simulink model "MotoTron_validation_IO_model_integration"  (R2018a)
settings: Solver=FixedStepDiscrete  StartTime=0.0  StopTime=10.0  RelTol=1e-3  EnableMultiTasking=on
undefined symbols (not defined in the file or in its folder): ECU565, motohawk_build_version, motohawk_trunc_name, motohawk_vardec_path
libraries: MotoHawk_lib x73, simulink x16, motohawk_examples_lib x1
(part 1 of 2)
settings Model: MotoHawkModelGUID=81168908-1F61-4548-B973-A09766F2E4F2  MotoHawkModelOpenTime=2019 4 16 12 38 3.57  MotoHawkBuildVersion=001  MotoHawkBuildStats=struct('TotalFLASH',{0},'TotalEEPROM',{0},'TotalRAM',{0},'AppFLASH',{0},'AppEEPROM',{0},'AppRAM',{0},'HeapRAM',{0},'BuildSuccessCount',{1},'BuildErrorCount',{0})  MotoHawkBuildDirectory=C:\Users\dhruv\OneDrive\Desktop\MEEM 5750\Project_Final5750\MotoTron_validation_IO_model_integration_Build  MotoHawkBuildInfo=struct('refmodel',{0},'model_name',{'MotoTron_validation_IO_model_2019'},'motohawk_version',{'2018a_sp2.2221'},'motohawk_component_version',{'0.0.8'},'motohawk_refmdl_version',{'0.0.1'},'matlab_version',{'9.4.0'},'build_version',{'000'},'module_type',{'ECU565-128'},'layout_type',{'DEV'},'enable_build',{1},'processor_family',{'PPC'},'processor_type',{'MPC565'},'toolchain_vendor',{'gcc-powerpc-eabi'},'toolchain_version',{'4.6.0'},'component',{0},'archive_file',{'PCM128.a'},'fptype',{0},'flash_size',{1048576},'ee_size',{8192},'ram_size',{36864},'decram_size',{4096},'eri_table0_rev',{12},'max_eri_table_size',{65535},'fgnd_base_period_ms',{5},'bgnd_base_period_ms',{50},'build_dir',{'D:\Slides\MotoTron_validation_IO_model_2019_Build'},'dll_name',{'MotoTron_validation_IO_model_2019_000'},'srz_name',{'MotoTron_validation_IO_model_2019_000'},'fgnd_stack_size',{3072},'fgnd_angle_stack_size',{0},'bgnd_stack_size',{2048},'idle_stack_size',{1024},'irq_stack_size',{1536},'irq_stack_margin',{153},'heap_size',{4096},'heap_margin',{409},'app_int_stack_size',{1024},'shutdown_stack_size',{1024},'use_target_os_config',{0},'num_cores_in_use',{1},'target_os',{'Classic ControlCore'},'install_dll_dir',{'C:\ECUFiles\TDBDLL'},'install_srz_dir',{'C:\ECUFiles\Programs'},'mingw_dir',{'C:\Program Files (x86)\Woodward\DevelopmentTools\Toolchains\GCC\win64-pe\4_7_1'},'motohawk_dir',{'C:\Program Files (x86)\Woodward\MCS\MotoHawk\2018a_sp2.2221'},'toolchain_dir',{'C:\Program Files (x86)\Woodward\DevelopmentTools\Toolchains\GCC\powerpc-eabi\4_6_0'},'matlab_root',{'C:\Program Files\MATLAB\R2018a'},'model_guid',{'030D1D23-8488-4897-A5F8-BE99CB1E4A09'},'build_guid',{'2DCC9D67-0315-4B80-8A59-7423BF9FA0F1'},'token_guid',{'26AE92E680E3264698612664E4C57D6C'})  MotoHawkModelSavedName=MotoTron_validation_IO_model_integration  MotoHawkModelElapsedTime=291694.622  MotoHawkBuildGUID=2DCC9D67-0315-4B80-8A59-7423BF9FA0F1  Creator=wzhouqua  LastModifiedBy=dhruv
settings ConfigSet: Description="This Simulink Configuration Set is preconfigured  for the MotoHawk target \"ECU565-128\"."
settings OptimizationCC: DefaultParameterBehavior=Inlined  InlineInvariantSignals=on  EnhancedBackFolding=on  InitFltsAndDblsToZero=on  NoFixptDivByZeroProtection=on  EfficientFloat2IntCast=on  LifeSpan=1
settings DebuggingCC: InheritedTsInSrcMsg=none  TasksWithSamePriorityMsg=none  ModelReferenceIOMismatchMessage=warning  SFUnexpectedBacktrackingDiag=warning  SFNoUnconditionalDefaultTransitionDiag=warning  SFExecutionAtInitializationDiag=none
settings HardwareCC: ProdBitPerPointer=32  ProdBitPerSizeT=32  ProdBitPerPtrDiffT=32  ProdLargestAtomicInteger=Integer  ProdIntDivRoundTo=Undefined  ProdEndianess=BigEndian  ProdWordSize=32  ProdHWDeviceType=Specified
settings ModelReferenceCC: UpdateModelReferenceTargets=IfOutOfDate  CheckModelReferenceTargetMessage=warning  ModelReferenceNumInstancesAllowed=Single
settings SFSimCC: MATLABDynamicMemAlloc=off
settings RTWCC: SystemTargetFile=motohawk_ert_rtw.tlc  MakeCommand=make_rtw_motohawk  TemplateMakefile=motohawk_ert_rtw.tmf  Description=MotoHawk(tm) Rapid Prototyping  GenerateReport=on  IncludeHyperlinkInReport=on  LaunchReport=on  GenerateTraceInfo=on  GenerateTraceReport=on  GenerateTraceReportSl=on  GenerateTraceReportSf=on  GenerateTraceReportEml=on
settings CodeAppCC: ForceParamTrailComments=on  IgnoreCustomStorageClasses=off  MaxIdLength=100  OperatorAnnotations=on  SimulinkDataObjDesc=on  SFDataObjDesc=on  MATLABFcnDesc=on  CustomSymbolStrType=$N$R$M  CustomSymbolStrField=$H$N$M  InsertBlockDesc=on  StateflowObjectComments=on  MATLABSourceComments=on  InternalIdentifier=Classic
settings STFCustomTargetCC: MultiwordTypeDef=User defined  MultiwordLength=0  IncludeMdlTerminateFcn=off  GeneratePreprocessorConditionals=Disable all  CombineOutputUpdateFcns=on  SuppressErrorStatus=on  ERTCustomFileBanners=on  SupportContinuousTime=off  SupportNonInlinedSFcns=off  RemoveResetFunc=on  MATLABClassNameForMDSCustomization=Simulink.SoftwareTarget.ERTCustomization  GRTInterface=off  SystemTargetFile=motohawk_ert_rtw.tlc
settings ERTTargetCC: MultiwordTypeDef=User defined  MultiwordLength=0  ParMdlRefBuildCompliant=off  CompOptLevelCompliant=off  ConcurrentExecutionCompliant=off  IncludeMdlTerminateFcn=off  GeneratePreprocessorConditionals=Disable all  SuppressErrorStatus=on  ModelStepFunctionPrototypeControlCompliant=off  CPPClassGenCompliant=off  UseToolchainInfoCompliant=off  InlinedParameterPlacement=NonHierarchical  ERTCustomFileTemplate=motohawk_file_process.tlc
settings ConfigComp: CovMetricSettings=dw  CovHtmlReporting=on  CovSaveCumulativeToWorkspaceVar=on  CovSaveSingleToWorkspaceVar=on  CovExternalEMLEnable=off

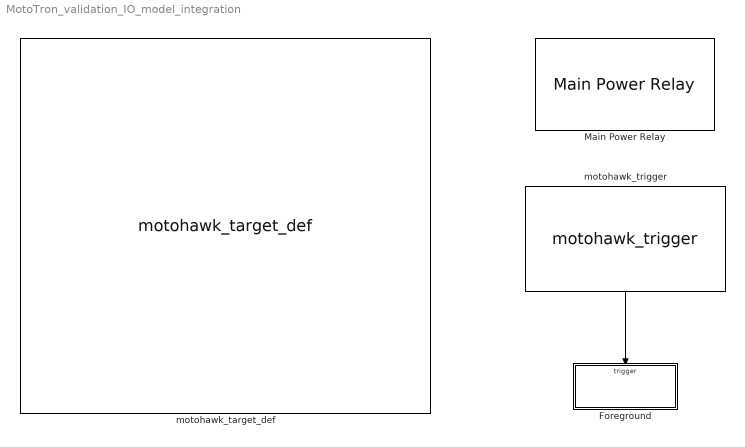
== system MotoTron_validation_IO_model_integration ==
  Foreground : Subsystem  InitFcn=data  TreatAsAtomicUnit=on
  Main Power Relay : motohawk_examples_lib/Main Power Relay Blocks/Main Power Relay  on_delay_count=2  off_delay_count=5  ecup_threshold=100  group='System | Main Power Relay'
      settings: SourceProductName=MotoHawk
  motohawk_target_def : MotoHawk_lib/motohawk_target_def  Priority=-65535  target=ECU565-128  layout=DEV  fptype=single (32 bits)  use_target_os_config=off  target_os=ControlCore  default_target_os=Classic ControlCore  fgnd_stack_size=3*1024  fgnd_angle_stack_size=0  bgnd_stack_size=2*1024  idle_stack_size=1024  irq_stack_size=1536  app_int_stack_size=1024  shutdown_stack_size=1024  heap_size=4*1024  show_margins=off  fgnd_stack_margin=(3*1024) * 0.1  fgnd_angle_stack_margin=0  bgnd_stack_margin=(2*1024) * 0.1  idle_stack_margin=(1024) * 0.1  irq_stack_margin=(1536) * 0.1  app_int_stack_margin=(1024) * 0.1  shutdown_stack_margin=(1024) * 0.1  heap_margin=(4*1024) * 0.1  comp_name=bdroot  comp_img='KVASER_CAN_USB.jpg'  comp_security=No Encryption  comp_build_pass='mhbuild'  comp_sim_pass='mhsim'  comp_multi=off  show_filenames=off  dll_name=motohawk_trunc_name(bdroot, ['_' motohawk_build_version], 50)  srz_name=motohawk_trunc_name(bdroot, ['_' motohawk_build_version], 50)  build_dir='.'  comp_dir='.'
      settings: SourceProductName=MotoHawk
  motohawk_trigger : MotoHawk_lib/Trigger Blocks/motohawk_trigger  Tag=Trigger  Priority=0  trig_name=[]  trigger=FGND_RTI_PERIODIC  priority_order=0  inherited=off  run_disabled=off  override_app_monitor=off  target=ECU565_128
      settings: SourceProductName=MotoHawk
  wires:
  motohawk_trigger/1 -> Foreground/Trigger

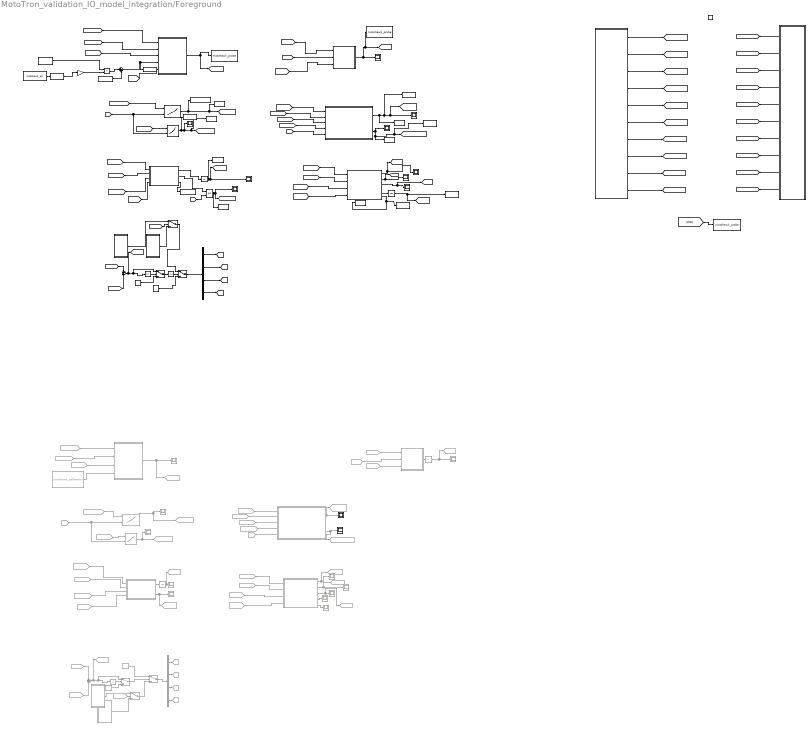
== system MotoTron_validation_IO_model_integration/Foreground ==
  note: Engine Start/Stop Model
  note: Torque Request
  note: Engine State Logic Model
  note: Blend Factor Lookup Tables
  note: StepperMotor
  note: Driving Mode Model
  note: E-Motor Start/Stop Model
  note: Blend Factor Lookup Tables
  note: Engine Start/Stop Model
  note: Driving Mode Model
  note: Engine State Logic Model
  note: StepperMotor
  note: E-Motor Start/Stop Model
  note: Torque Request
  function : TriggerPort  TriggerType=function-call  VariantControl=Variant
  2-D Lookup Table : Lookup_n-D  Commented=on  BreakpointsForDimension1=Engine_Blend_Factor(2:end,1)  BreakpointsForDimension2=Engine_Blend_Factor(1,2:end)  Table=Engine_Blend_Factor(2:end,2:end)  InternalRulePriority=Speed  RndMeth=Simplest  InputSameDT=on
  2-D Lookup Table1 : Lookup_n-D  InitFcn=data  BreakpointsForDimension1=Engine_Blend_Factor(2:end,1)  BreakpointsForDimension2=Engine_Blend_Factor(1,2:end)  Table=Engine_Blend_Factor(2:end,2:end)  InternalRulePriority=Speed  RndMeth=Simplest  InputSameDT=on
  Abs : Abs  Commented=on
  Abs1 : Abs
  Abs2 : Abs
  Actuator : Subsystem
  CCW : Subsystem  Commented=on
  CCW1 : Subsystem
  CW : Subsystem  Commented=on
  CW1 : Subsystem
  Cast : DataTypeConversion  OutDataTypeStr=double
  Chart : Stateflow chart  Commented=on  TreatAsAtomicUnit=on
  Chart1 : Stateflow chart  Commented=on  TreatAsAtomicUnit=on
  Chart2 : Stateflow chart  TreatAsAtomicUnit=on
  Chart3 : Stateflow chart  TreatAsAtomicUnit=on
  Constant : Constant  Commented=on  Value=0
  Constant1 : Constant  Commented=on  Value=0
  Constant2 : Constant  Value=0
  Constant3 : Constant  Value=0
  Demux : Demux  Commented=on
  Demux1 : Demux
  "Engine State " : Stateflow chart  Commented=on  TreatAsAtomicUnit=on
  Engine State 1 : Stateflow chart  TreatAsAtomicUnit=on
  From : From  Commented=on  GotoTag=Vehicle_Speed
  From11 : From  Commented=on  GotoTag=Vehicle_Speed
  From12 : From  Commented=on  GotoTag=motorblendfactor
  From13 : From  Commented=on  GotoTag=drivingmode
  From14 : From  Commented=on  GotoTag=engineblendfactor
  From15 : From  Commented=on  GotoTag=motorblendfactor
  From16 : From  Commented=on  GotoTag=drivingmode
  From17 : From  Commented=on  GotoTag=Engine_State
  From18 : From  Commented=on  GotoTag=PPS1
  From19 : From  Commented=on  GotoTag=engineblendfactor
  From20 : From  Commented=on  GotoTag=drivingmode
  From21 : From  Commented=on  GotoTag=Engine_State
  From22 : From  Commented=on  GotoTag=Engine_On_Switch
  From23 : From  Commented=on  GotoTag=Motor_On_Switch
  From24 : From  Commented=on  GotoTag=Vehicle_Speed
  From25 : From  Commented=on  GotoTag=Engine_RPM
  From26 : From  Commented=on  GotoTag=Crank_Switch
  From27 : From  Commented=on  GotoTag=PPS1
  From28 : From  Commented=on  GotoTag=Crank_Switch
  From29 : From  Commented=on  GotoTag=Forward_Switch
  From30 : From  Commented=on  GotoTag=Reverse_Switch
  From31 : From  Commented=on  GotoTag=enginethrottle
  From32 : From  Commented=on  GotoTag=TPS
  From33 : From  Commented=on  GotoTag=Engine_Kill
  From35 : From  Commented=on  GotoTag=difference
  Gain : Gain  Gain=5/1023
  Goto10 : Goto  Commented=on  GotoTag=Engine_State
  Goto11 : Goto  Commented=on  GotoTag=engineblendfactor
  Goto12 : Goto  Commented=on  GotoTag=motorblendfactor
  Goto13 : Goto  Commented=on  GotoTag=E_Motor_Toruqe_Request
  Goto14 : Goto  Commented=on  GotoTag=Forward
  Goto15 : Goto  Commented=on  GotoTag=enginethrottle
  Goto16 : Goto  Commented=on  GotoTag=Coil_4
  Goto17 : Goto  Commented=on  GotoTag=Coil_1
  Goto18 : Goto  Commented=on  GotoTag=Coil_2
  Goto19 : Goto  Commented=on  GotoTag=Coil_3
  Goto20 : Goto  Commented=on  GotoTag=Engine_Crank
  Goto21 : Goto  Commented=on  GotoTag=Engine_Kill
  Goto22 : Goto  Commented=on  GotoTag=Reverse
  Goto23 : Goto  Commented=on  GotoTag=E_motor_on
  Goto24 : Goto  Commented=on  GotoTag=difference
  Goto25 : Goto  Commented=on  GotoTag=drivingmode
  MATLAB Function : MATLAB Function  Commented=on  TreatAsAtomicUnit=on
  MATLAB Function1 : MATLAB Function  Commented=on  TreatAsAtomicUnit=on
  MATLAB Function2 : MATLAB Function  TreatAsAtomicUnit=on
  MATLAB Function3 : MATLAB Function  TreatAsAtomicUnit=on
  "Motor Blend Factor " : Lookup_n-D  Commented=on  BreakpointsForDimension1=Motor_Blend_Factor(2:end,1)  BreakpointsForDimension2=Motor_Blend_Factor(1,2:end)  Table=Motor_Blend_Factor(2:end,2:end)  InternalRulePriority=Speed  RndMeth=Simplest  InputSameDT=on
  Motor Blend Factor 1 : Lookup_n-D  BreakpointsForDimension1=Motor_Blend_Factor(2:end,1)  BreakpointsForDimension2=Motor_Blend_Factor(1,2:end)  Table=Motor_Blend_Factor(2:end,2:end)  InternalRulePriority=Speed  RndMeth=Simplest  InputSameDT=on
  OR : Logic  Operator=OR  IconShape=distinctive  AllPortsSameDT=off  OutDataTypeStr=boolean
  Product : Product
  Scope{,1,4..12} (11 alike) : Scope  Commented=on
  Scope{2..3,14..15,21..22,24..28} (11 alike) : Scope
  Sensors : Subsystem
  Sum : Sum  Commented=on  Inputs=+-
  Sum1 : Sum  Inputs=+-
  Sum2 : Sum  Inputs=|++
  Switch : Switch  Commented=on  Criteria=u2 > Threshold  Threshold=1
  Switch1 : Switch  Commented=on  Criteria=u2 ~= 0
  Switch2 : Switch  Commented=on  Criteria=u2 > Threshold
  Switch3 : Switch  Criteria=u2 > Threshold  Threshold=1
  Switch4 : Switch  Criteria=u2 > Threshold
  Switch5 : Switch  Criteria=u2 > Threshold
  To Workspace12 : ToWorkspace  VariableName=motorkill  SaveFormat=Timeseries  SampleTime=-1
  To Workspace2 : ToWorkspace  VariableName=engineblend  SaveFormat=Timeseries  SampleTime=-1
  To Workspace3 : ToWorkspace  VariableName=motorblend  SaveFormat=Timeseries  SampleTime=-1
  To Workspace4 : ToWorkspace  VariableName=enginetorque  SaveFormat=Timeseries  SampleTime=-1
  To Workspace5 : ToWorkspace  VariableName=motortorque  SaveFormat=Timeseries  SampleTime=-1
  To Workspace6 : ToWorkspace  VariableName=enginekill  SaveFormat=Timeseries  SampleTime=-1
  To Workspace7 : ToWorkspace  VariableName=enginecrank  SaveFormat=Timeseries  SampleTime=-1
  Unit Delay : UnitDelay  Commented=on  SampleTime=-1
  Unit Delay1 : UnitDelay  Commented=on  SampleTime=-1
  Unit Delay2 : UnitDelay  SampleTime=-1
  Unit Delay3 : UnitDelay  SampleTime=-1
  motohawk_ain : MotoHawk_lib/Analog I//O Blocks/motohawk_ain  res_name='SOC'  text_resource=AN9M  code_resource=NONE  val_resource=-1  target=ECU565-128  resource_enum_str=(None)=-1,ECUP=53,DRVP=54,XDRP=55,AN1M=56,AN2M=57,AN3M=58,AN4M=59,AN5M=60,AN6M=61,AN7M=62,AN8M=63,AN9M=64,AN10M=65,AN11M=66,AN12M=67,AN13M=68,AN14M=69,AN15M=70,AN16M=71,AN17M=72,AN18M=73,AN19M=74,AN20M=75,AN21M=76,AN22M=77,AN23M=78,AN24M=79,AN25M=80,AN26M=81,AN27M=82,AN28M=83,AN29M=84,AN30M=85,AN31M=86,AN32M=87,AN33M=88,AN34M=89,O2A=90,O2B=91,XDRP_B=92,REF_14V=143  altref=5V Reference  typ=uint16  num_adc_bits=10  use_stat=off  use_vardec=off  nam='RTD1_MW'  read_level=1  write_level=1  group='System | I/O Pins | Inputs Config'
      settings: SourceProductName=MotoHawk
  motohawk_calibration : MotoHawk_lib/Calibration & Probing Blocks/motohawk_calibration  Commented=on  nam='MyCal'  val=0.5  storage=Calibration  show_more=off  name_source=Use Parameter  data_type=Inherit from 'Default Value'  read_level=1  write_level=1  ovr_cals=on  view_as=Number  enum_struct={'Disabled', 'Enabled'}  vector_style=Wide Row  use_help_units=off  help=''  units=''  use_header_enum=off  row_header_enum={}  col_header_enum={}  use_min_max=off  min_val=-inf  max_val=inf  use_precision=off  precision=''  gain=1  offset=0  exp=1  use_mototune_group=off  mototune_group=motohawk_vardec_path(gcb)  data_stores=motohawk_sfun_calibration_data_stores
      settings: SourceProductName=MotoHawk
  motohawk_calibration1 : MotoHawk_lib/Calibration & Probing Blocks/motohawk_calibration  nam='SOCGain'  val=0  storage=Calibration  show_more=off  name_source=Use Parameter  data_type=Inherit from 'Default Value'  read_level=1  write_level=1  ovr_cals=on  view_as=Number  enum_struct={'Disabled', 'Enabled'}  vector_style=Wide Row  use_help_units=off  help=''  units=''  use_header_enum=off  row_header_enum={}  col_header_enum={}  use_min_max=off  min_val=-inf  max_val=inf  use_precision=off  precision=''  gain=1  offset=0  exp=1  use_mototune_group=off  mototune_group=motohawk_vardec_path(gcb)  data_stores=motohawk_sfun_calibration_data_stores
      settings: SourceProductName=MotoHawk
  motohawk_calibration2 : MotoHawk_lib/Calibration & Probing Blocks/motohawk_calibration  nam='SOCOffset'  val=0  storage=Calibration  show_more=off  name_source=Use Parameter  data_type=Inherit from 'Default Value'  read_level=1  write_level=1  ovr_cals=on  view_as=Number  enum_struct={'Disabled', 'Enabled'}  vector_style=Wide Row  use_help_units=off  help=''  units=''  use_header_enum=off  row_header_enum={}  col_header_enum={}  use_min_max=off  min_val=-inf  max_val=inf  use_precision=off  precision=''  gain=1  offset=0  exp=1  use_mototune_group=off  mototune_group=motohawk_vardec_path(gcb)  data_stores=motohawk_sfun_calibration_data_stores
      settings: SourceProductName=MotoHawk
  motohawk_probe : MotoHawk_lib/Calibration & Probing Blocks/motohawk_probe  nam='Probe'  show_more=off  name_source=Use Parameter  read_level=1  view_as=Number  enum_struct={'Disabled', 'Enabled'}  vector_style=Wide Row  use_help_units=off  help=''  units=''  use_header_enum=off  row_header_enum={}  col_header_enum={}  use_min_max=off  min_val=-inf  max_val=inf  use_precision=off  precision=''  gain=1  offset=0  exp=1  use_mototune_group=off  mototune_group=motohawk_vardec_path(gcb)
      settings: SourceProductName=MotoHawk
  motohawk_probe1 : MotoHawk_lib/Calibration & Probing Blocks/motohawk_probe  nam='Autocrank_Validation'  show_more=off  name_source=Use Parameter  read_level=1  view_as=Number  enum_struct={'Disabled', 'Enabled'}  vector_style=Wide Row  use_help_units=off  help=''  units=''  use_header_enum=off  row_header_enum={}  col_header_enum={}  use_min_max=off  min_val=-inf  max_val=inf  use_precision=off  precision=''  gain=1  offset=0  exp=1  use_mototune_group=off  mototune_group=motohawk_vardec_path(gcb)
      settings: SourceProductName=MotoHawk
  motohawk_probe10 : MotoHawk_lib/Calibration & Probing Blocks/motohawk_probe  nam='motortorquerequest'  show_more=off  name_source=Use Parameter  read_level=1  view_as=Number  enum_struct={'Disabled', 'Enabled'}  vector_style=Wide Row  use_help_units=off  help=''  units=''  use_header_enum=off  row_header_enum={}  col_header_enum={}  use_min_max=off  min_val=-inf  max_val=inf  use_precision=off  precision=''  gain=1  offset=0  exp=1  use_mototune_group=off  mototune_group=motohawk_vardec_path(gcb)
      settings: SourceProductName=MotoHawk
  motohawk_probe2 : MotoHawk_lib/Calibration & Probing Blocks/motohawk_probe  nam='Autocrank'  show_more=off  name_source=Use Parameter  read_level=1  view_as=Number  enum_struct={'Disabled', 'Enabled'}  vector_style=Wide Row  use_help_units=off  help=''  units=''  use_header_enum=off  row_header_enum={}  col_header_enum={}  use_min_max=off  min_val=-inf  max_val=inf  use_precision=off  precision=''  gain=1  offset=0  exp=1  use_mototune_group=off  mototune_group=motohawk_vardec_path(gcb)
      settings: SourceProductName=MotoHawk
  motohawk_probe3 : MotoHawk_lib/Calibration & Probing Blocks/motohawk_probe  nam='Motorkill'  show_more=off  name_source=Use Parameter  read_level=1  view_as=Number  enum_struct={'Disabled', 'Enabled'}  vector_style=Wide Row  use_help_units=off  help=''  units=''  use_header_enum=off  row_header_enum={}  col_header_enum={}  use_min_max=off  min_val=-inf  max_val=inf  use_precision=off  precision=''  gain=1  offset=0  exp=1  use_mototune_group=off  mototune_group=motohawk_vardec_path(gcb)
      settings: SourceProductName=MotoHawk
  motohawk_probe4 : MotoHawk_lib/Calibration & Probing Blocks/motohawk_probe  nam='DriveMode'  show_more=off  name_source=Use Parameter  read_level=1  view_as=Number  enum_struct={'Disabled', 'Enabled'}  vector_style=Wide Row  use_help_units=off  help=''  units=''  use_header_enum=off  row_header_enum={}  col_header_enum={}  use_min_max=off  min_val=-inf  max_val=inf  use_precision=off  precision=''  gain=1  offset=0  exp=1  use_mototune_group=off  mototune_group=motohawk_vardec_path(gcb)
      settings: SourceProductName=MotoHawk
  motohawk_probe5 : MotoHawk_lib/Calibration & Probing Blocks/motohawk_probe  nam='SOC'  show_more=off  name_source=Use Parameter  read_level=1  view_as=Number  enum_struct={'Disabled', 'Enabled'}  vector_style=Wide Row  use_help_units=off  help=''  units=''  use_header_enum=off  row_header_enum={}  col_header_enum={}  use_min_max=off  min_val=-inf  max_val=inf  use_precision=off  precision=''  gain=1  offset=0  exp=1  use_mototune_group=off  mototune_group=motohawk_vardec_path(gcb)
      settings: SourceProductName=MotoHawk
  motohawk_probe6 : MotoHawk_lib/Calibration & Probing Blocks/motohawk_probe  nam='EngineState'  show_more=off  name_source=Use Parameter  read_level=1  view_as=Number  enum_struct={'Disabled', 'Enabled'}  vector_style=Wide Row  use_help_units=off  help=''  units=''  use_header_enum=off  row_header_enum={}  col_header_enum={}  use_min_max=off  min_val=-inf  max_val=inf  use_precision=off  precision=''  gain=1  offset=0  exp=1  use_mototune_group=off  mototune_group=motohawk_vardec_path(gcb)
      settings: SourceProductName=MotoHawk
  motohawk_probe7 : MotoHawk_lib/Calibration & Probing Blocks/motohawk_probe  nam='enginetorquerequest'  show_more=off  name_source=Use Parameter  read_level=1  view_as=Number  enum_struct={'Disabled', 'Enabled'}  vector_style=Wide Row  use_help_units=off  help=''  units=''  use_header_enum=off  row_header_enum={}  col_header_enum={}  use_min_max=off  min_val=-inf  max_val=inf  use_precision=off  precision=''  gain=1  offset=0  exp=1  use_mototune_group=off  mototune_group=motohawk_vardec_path(gcb)
      settings: SourceProductName=MotoHawk
  motohawk_probe8 : MotoHawk_lib/Calibration & Probing Blocks/motohawk_probe  nam='EngineBlendFactor'  show_more=off  name_source=Use Parameter  read_level=1  view_as=Number  enum_struct={'Disabled', 'Enabled'}  vector_style=Wide Row  use_help_units=off  help=''  units=''  use_header_enum=off  row_header_enum={}  col_header_enum={}  use_min_max=off  min_val=-inf  max_val=inf  use_precision=off  precision=''  gain=1  offset=0  exp=1  use_mototune_group=off  mototune_group=motohawk_vardec_path(gcb)
      settings: SourceProductName=MotoHawk
  motohawk_probe9 : MotoHawk_lib/Calibration & Probing Blocks/motohawk_probe  nam='Coil2'  show_more=off  name_source=Use Parameter  read_level=1  view_as=Number  enum_struct={'Disabled', 'Enabled'}  vector_style=Wide Row  use_help_units=off  help=''  units=''  use_header_enum=off  row_header_enum={}  col_header_enum={}  use_min_max=off  min_val=-inf  max_val=inf  use_precision=off  precision=''  gain=1  offset=0  exp=1  use_mototune_group=off  mototune_group=motohawk_vardec_path(gcb)
      settings: SourceProductName=MotoHawk
  wires:
  [Engine_Crank] -> Actuator/1(In1)
  [Forward] -> Actuator/2(In2)
  [Reverse] -> Actuator/3(In3)
  [E_motor_on] -> Actuator/4(In4)
  [Engine_Kill] -> Actuator/5(In5)
  [Coil_1] -> Actuator/6(In6)
  [Coil_2] -> Actuator/7(In7)
  [Coil_3] -> Actuator/8(In8)
  [Coil_4] -> Actuator/9(In9)
  [E_Motor_Toruqe_Request] -> Actuator/10(In10)
  Sensors/6(Out6) -> [PPS1]
  Sensors/1(Out1) -> [Crank_Switch]
  Sensors/2(Out2) -> [Engine_On_Switch]
  Sensors/3(Out3) -> [Motor_On_Switch]
  Sensors/4(Out4) -> [Forward_Switch]
  Sensors/5(Out5) -> [Reverse_Switch]
  Sensors/7(Out7) -> [PPS2]
  Sensors/8(Out8) -> [TPS]
  Sensors/9(Out9) -> [Vehicle_Speed]
  Sensors/10(Out10) -> [Engine_RPM]
  From20/1 -> MATLAB Function/2(drivingmode)
  From19/1 -> MATLAB Function/1(engineblendfactor)
  From17/1 -> Chart1/4(EngineState)
  From18/1 -> Chart1/5(APP)
  Chart1/2(motortorquerequest) -> Goto13/1, Scope3/1
  MATLAB Function/2(enginecrank) -> Goto20/1, Scope7/1
  From11/1 -> "Motor Blend Factor "/1
  Chart1/1(enginetorquerequest) -> Scope2/1, Goto15/1
  From16/1 -> Chart1/3(DrivingMode)
  From27/1 -> "Motor Blend Factor "/2, 2-D Lookup Table/2
  From14/1 -> Chart1/1(EngineBlendFactor)
  "Motor Blend Factor "/1 -> Scope5/1, Goto12/1
  From21/1 -> MATLAB Function/3(Engine_State)
  2-D Lookup Table/1 -> Goto11/1, Scope4/1
  From15/1 -> Chart1/2(MotorBlendFactor)
  From/1 -> 2-D Lookup Table/1
  Demux/4 -> Goto16/1
  Sum/1 -> Goto24/1, Switch/1, Abs/1
  Abs/1 -> Switch/2
  Demux/1 -> Goto17/1
  Demux/3 -> Goto19/1
  Demux/2 -> Goto18/1
  From25/1 -> "Engine State "/1(RPM)
  From26/1 -> "Engine State "/3(crank)
  From28/1 -> MATLAB Function/4(crankswitch)
  From31/1 -> Sum/1
  From32/1 -> Sum/2
  From33/1 -> "Engine State "/2(kill)
  "Engine State "/1(engine_state) -> Unit Delay/1
  Unit Delay/1 -> Goto10/1, Scope1/1
  MATLAB Function/1(enginekill) -> Unit Delay1/1
  Unit Delay1/1 -> Goto21/1, Scope6/1
  Chart/1(drive_mode) -> Goto25/1, Scope/1
  motohawk_calibration/1 -> Chart/4(SOC)
  From22/1 -> Chart/1(Eon)
  From23/1 -> Chart/2(mon)
  From24/1 -> Chart/3(velocity)
  MATLAB Function1/2(forward) -> Goto14/1, Scope9/1
  MATLAB Function1/5(motorkill) -> Scope12/1
  From30/1 -> MATLAB Function1/4(reverseswitch)
  MATLAB Function1/4(autocrank) -> Scope11/1
  MATLAB Function1/3(reverse) -> Goto22/1, Scope10/1
  From12/1 -> MATLAB Function1/1(motorblendfactor)
  From29/1 -> MATLAB Function1/3(forwardswitch)
  MATLAB Function1/1(emotoron) -> Goto23/1, Scope8/1
  From13/1 -> MATLAB Function1/2(drivingmode)
  [PPS2] -> motohawk_probe/1
  Constant/1 -> Switch/3
  Switch/1 -> Switch1/2
  Constant1/1 -> Switch1/1
  CW/1(Out1) -> Switch2/1
  CCW/1(Out1) -> Switch2/3
  Switch2/1 -> Switch1/3
  From35/1 -> Switch2/2
  Switch1/1 -> Demux/1
  Unit Delay3/1 -> motohawk_probe2/1, [autocrank]
  Switch5/1 -> Switch4/1
  [Engine_State] -> MATLAB Function2/3(Engine_State)
  [drivingmode] -> MATLAB Function2/2(drivingmode)
  [Vehicle_Speed] -> Motor Blend Factor 1/1
  [engineblendfactor] -> MATLAB Function2/1(engineblendfactor)
  CCW1/1(Out1) -> Switch5/3
  [autocrank] -> Chart2/5(autocrank)
  [autocrank] -> OR/2
  Constant2/1 -> Switch4/3
  [Crank_Switch] -> Engine State 1/3(crank)
  Engine State 1/1(engine_state) -> motohawk_probe6/1, [Engine_State], Scope14/1
  Chart3/2(motortorquerequest) -> Scope22/1, motohawk_probe10/1, [E_Motor_Toruqe_Request], To Workspace5/1
  [Vehicle_Speed] -> Chart2/3(velocity)
  [PPS1] -> Motor Blend Factor 1/2, 2-D Lookup Table1/2
  [difference] -> Switch5/2
  Constant3/1 -> Switch3/3
  MATLAB Function3/2(forward) -> [Forward], Scope28/1
  Demux1/1 -> [Coil_1]
  Sum1/1 -> [difference], Switch3/1, Abs1/1
  Abs1/1 -> Switch3/2
  Demux1/2 -> [Coil_2]
  Demux1/3 -> [Coil_3]
  OR/1 -> To Workspace7/1, [Engine_Crank], Scope26/1
  [Engine_Kill] -> Engine State 1/2(kill)
  Unit Delay2/1 -> To Workspace6/1, [Engine_Kill], Scope25/1
  MATLAB Function3/4(autocrank) -> Unit Delay3/1
  MATLAB Function3/1(emotoron) -> [E_motor_on], Scope27/1
  MATLAB Function3/5(motorkill) -> motohawk_probe3/1, To Workspace12/1
  [motorblendfactor] -> Chart3/2(MotorBlendFactor)
  MATLAB Function2/1(enginekill) -> Unit Delay2/1
  CW1/1(Out1) -> Switch5/1
  MATLAB Function3/3(reverse) -> [Reverse], Scope15/1
  Switch4/1 -> Demux1/1
  Chart3/1(enginetorquerequest) -> motohawk_probe7/1, [enginethrottle], Scope21/1, To Workspace4/1
  [Engine_State] -> Chart3/4(EngineState)
  [Motor_On_Switch] -> Chart2/2(mon)
  Demux1/4 -> [Coil_4]
  [Engine_RPM] -> Engine State 1/1(RPM)
  Switch3/1 -> Abs2/1
  Abs2/1 -> Switch4/2
  Motor Blend Factor 1/1 -> motohawk_probe9/1, Scope24/1, [motorblendfactor], To Workspace3/1
  [drivingmode] -> Chart3/3(DrivingMode)
  [PPS1] -> Chart3/5(APP)
  MATLAB Function2/2(enginecrank) -> OR/1
  [Vehicle_Speed] -> 2-D Lookup Table1/1
  Chart2/1(drive_mode) -> motohawk_probe4/1, [drivingmode]
  [engineblendfactor] -> Chart3/1(EngineBlendFactor)
  [Engine_On_Switch] -> Chart2/1(Eon)
  2-D Lookup Table1/1 -> motohawk_probe8/1, [engineblendfactor], To Workspace2/1
  motohawk_calibration1/1 -> Product/1
  motohawk_ain/1 -> Cast/1
  Product/1 -> Sum2/1
  motohawk_calibration2/1 -> Sum2/2
  Sum2/1 -> motohawk_probe5/1, Chart2/4(SOC)
  [enginethrottle] -> Sum1/1
  [TPS] -> Sum1/2
  [Crank_Switch] -> MATLAB Function2/4(crankswitch)
  [Forward_Switch] -> MATLAB Function3/3(forwardswitch)
  [drivingmode] -> MATLAB Function3/2(drivingmode)
  [motorblendfactor] -> MATLAB Function3/1(motorblendfactor)
  [Reverse_Switch] -> MATLAB Function3/4(reverseswitch)
  Cast/1 -> Gain/1
  Gain/1 -> Product/2
  MATLAB Function2/3(auto_crank) -> motohawk_probe1/1

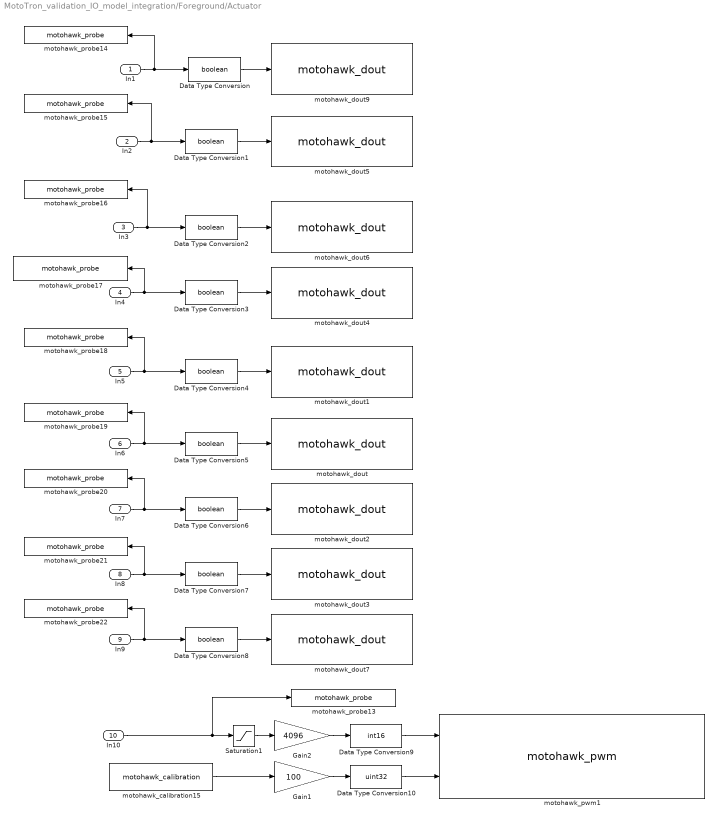
== system MotoTron_validation_IO_model_integration/Foreground/Actuator ==
  In1 : Inport
  In2 : Inport  Port=2
  In3 : Inport  Port=3
  In4 : Inport  Port=4
  In5 : Inport  Port=5
  In6 : Inport  Port=6
  In7 : Inport  Port=7
  In8 : Inport  Port=8
  In9 : Inport  Port=9
  In10 : Inport  Port=10
  Data Type Conversion{,1..8} (9 alike) : DataTypeConversion  OutDataTypeStr=boolean
  Data Type Conversion10 : DataTypeConversion  OutDataTypeStr=uint32
  Data Type Conversion9 : DataTypeConversion  OutDataTypeStr=int16
  Gain1 : Gain  Gain=100  OutDataTypeStr=Inherit: Inherit via back propagation
  Gain2 : Gain  Gain=4096  OutDataTypeStr=Inherit: Inherit via back propagation
  Saturation1 : Saturate  UpperLimit=0.36  LowerLimit=0
  motohawk_calibration15 : MotoHawk_lib/Calibration & Probing Blocks/motohawk_calibration  nam='Throttle_Frequency'  val=10000  storage=Calibration  show_more=on  name_source=Use Parameter  data_type=Inherit via back propagation  read_level=1  write_level=1  ovr_cals=on  view_as=Number  enum_struct={'Disabled', 'Enabled'}  vector_style=Wide Row  use_help_units=off  help=''  units=''  use_header_enum=off  row_header_enum={}  col_header_enum={}  use_min_max=off  min_val=-inf  max_val=inf  use_precision=off  precision=''  gain=1  offset=0  exp=1  use_mototune_group=off  mototune_group=motohawk_vardec_path(gcb)  data_stores=motohawk_sfun_calibration_data_stores
      settings: SourceProductName=MotoHawk
  motohawk_dout : MotoHawk_lib/Digital I//O Blocks/motohawk_dout  resource_name=[]  text_resource=LSD5  target=ECU565-128  use_diag=off  use_vardec=off  nam='DOUT'  read_level=1  write_level=1  group='System | I/O Pins | Outputs Config'
      settings: SourceProductName=MotoHawk
  motohawk_dout1 : MotoHawk_lib/Digital I//O Blocks/motohawk_dout  resource_name=[]  text_resource=LSD9  target=ECU565-128  use_diag=off  use_vardec=off  nam='DOUT'  read_level=1  write_level=1  group='System | I/O Pins | Outputs Config'
      settings: SourceProductName=MotoHawk
  motohawk_dout2 : MotoHawk_lib/Digital I//O Blocks/motohawk_dout  resource_name=[]  text_resource=LSD6  target=ECU565-128  use_diag=off  use_vardec=off  nam='DOUT'  read_level=1  write_level=1  group='System | I/O Pins | Outputs Config'
      settings: SourceProductName=MotoHawk
  motohawk_dout3 : MotoHawk_lib/Digital I//O Blocks/motohawk_dout  resource_name=[]  text_resource=LSD7  target=ECU565-128  use_diag=off  use_vardec=off  nam='DOUT'  read_level=1  write_level=1  group='System | I/O Pins | Outputs Config'
      settings: SourceProductName=MotoHawk
  motohawk_dout4 : MotoHawk_lib/Digital I//O Blocks/motohawk_dout  resource_name=[]  text_resource=LSD4  target=ECU565-128  use_diag=off  use_vardec=off  nam='DOUT'  read_level=1  write_level=1  group='System | I/O Pins | Outputs Config'
      settings: SourceProductName=MotoHawk
  motohawk_dout5 : MotoHawk_lib/Digital I//O Blocks/motohawk_dout  resource_name=[]  text_resource=LSD2  target=ECU565-128  use_diag=off  use_vardec=off  nam='DOUT'  read_level=1  write_level=1  group='System | I/O Pins | Outputs Config'
      settings: SourceProductName=MotoHawk
  motohawk_dout6 : MotoHawk_lib/Digital I//O Blocks/motohawk_dout  resource_name=[]  text_resource=LSD3  target=ECU565-128  use_diag=off  use_vardec=off  nam='DOUT'  read_level=1  write_level=1  group='System | I/O Pins | Outputs Config'
      settings: SourceProductName=MotoHawk
  motohawk_dout7 : MotoHawk_lib/Digital I//O Blocks/motohawk_dout  resource_name=[]  text_resource=LSD8  target=ECU565-128  use_diag=off  use_vardec=off  nam='DOUT'  read_level=1  write_level=1  group='System | I/O Pins | Outputs Config'
      settings: SourceProductName=MotoHawk
  motohawk_dout9 : MotoHawk_lib/Digital I//O Blocks/motohawk_dout  resource_name=[]  text_resource=LSD1  target=ECU565-128  use_diag=off  use_vardec=off  nam='DOUT'  read_level=1  write_level=1  group='System | I/O Pins | Outputs Config'
      settings: SourceProductName=MotoHawk
  motohawk_probe13 : MotoHawk_lib/Calibration & Probing Blocks/motohawk_probe  nam='E_Motor_Toruqe_Request'  show_more=off  name_source=Use Parameter  read_level=1  view_as=Number  enum_struct={'Disabled', 'Enabled'}  vector_style=Wide Row  use_help_units=off  help=''  units=''  use_header_enum=off  row_header_enum={}  col_header_enum={}  use_min_max=off  min_val=-inf  max_val=inf  use_precision=off  precision=''  gain=1  offset=0  exp=1  use_mototune_group=off  mototune_group=motohawk_vardec_path(gcb)
      settings: SourceProductName=MotoHawk
  motohawk_probe14 : MotoHawk_lib/Calibration & Probing Blocks/motohawk_probe  nam='Engine_Crank'  show_more=off  name_source=Use Parameter  read_level=1  view_as=Number  enum_struct={'Disabled', 'Enabled'}  vector_style=Wide Row  use_help_units=off  help=''  units=''  use_header_enum=off  row_header_enum={}  col_header_enum={}  use_min_max=off  min_val=-inf  max_val=inf  use_precision=off  precision=''  gain=1  offset=0  exp=1  use_mototune_group=off  mototune_group=motohawk_vardec_path(gcb)
      settings: SourceProductName=MotoHawk
  motohawk_probe15 : MotoHawk_lib/Calibration & Probing Blocks/motohawk_probe  nam='Foward'  show_more=off  name_source=Use Parameter  read_level=1  view_as=Number  enum_struct={'Disabled', 'Enabled'}  vector_style=Wide Row  use_help_units=off  help=''  units=''  use_header_enum=off  row_header_enum={}  col_header_enum={}  use_min_max=off  min_val=-inf  max_val=inf  use_precision=off  precision=''  gain=1  offset=0  exp=1  use_mototune_group=off  mototune_group=motohawk_vardec_path(gcb)
      settings: SourceProductName=MotoHawk
  motohawk_probe16 : MotoHawk_lib/Calibration & Probing Blocks/motohawk_probe  nam='Reverse'  show_more=off  name_source=Use Parameter  read_level=1  view_as=Number  enum_struct={'Disabled', 'Enabled'}  vector_style=Wide Row  use_help_units=off  help=''  units=''  use_header_enum=off  row_header_enum={}  col_header_enum={}  use_min_max=off  min_val=-inf  max_val=inf  use_precision=off  precision=''  gain=1  offset=0  exp=1  use_mototune_group=off  mototune_group=motohawk_vardec_path(gcb)
      settings: SourceProductName=MotoHawk
  motohawk_probe17 : MotoHawk_lib/Calibration & Probing Blocks/motohawk_probe  nam='E_Motor_On'  show_more=off  name_source=Use Parameter  read_level=1  view_as=Number  enum_struct={'Disabled', 'Enabled'}  vector_style=Wide Row  use_help_units=off  help=''  units=''  use_header_enum=off  row_header_enum={}  col_header_enum={}  use_min_max=off  min_val=-inf  max_val=inf  use_precision=off  precision=''  gain=1  offset=0  exp=1  use_mototune_group=off  mototune_group=motohawk_vardec_path(gcb)
      settings: SourceProductName=MotoHawk
  motohawk_probe18 : MotoHawk_lib/Calibration & Probing Blocks/motohawk_probe  nam='Engine_Kill'  show_more=off  name_source=Use Parameter  read_level=1  view_as=Number  enum_struct={'Disabled', 'Enabled'}  vector_style=Wide Row  use_help_units=off  help=''  units=''  use_header_enum=off  row_header_enum={}  col_header_enum={}  use_min_max=off  min_val=-inf  max_val=inf  use_precision=off  precision=''  gain=1  offset=0  exp=1  use_mototune_group=off  mototune_group=motohawk_vardec_path(gcb)
      settings: SourceProductName=MotoHawk
  motohawk_probe19 : MotoHawk_lib/Calibration & Probing Blocks/motohawk_probe  nam='Coil_1'  show_more=off  name_source=Use Parameter  read_level=1  view_as=Number  enum_struct={'Disabled', 'Enabled'}  vector_style=Wide Row  use_help_units=off  help=''  units=''  use_header_enum=off  row_header_enum={}  col_header_enum={}  use_min_max=off  min_val=-inf  max_val=inf  use_precision=off  precision=''  gain=1  offset=0  exp=1  use_mototune_group=off  mototune_group=motohawk_vardec_path(gcb)
      settings: SourceProductName=MotoHawk
  motohawk_probe20 : MotoHawk_lib/Calibration & Probing Blocks/motohawk_probe  nam='Coil_2'  show_more=off  name_source=Use Parameter  read_level=1  view_as=Number  enum_struct={'Disabled', 'Enabled'}  vector_style=Wide Row  use_help_units=off  help=''  units=''  use_header_enum=off  row_header_enum={}  col_header_enum={}  use_min_max=off  min_val=-inf  max_val=inf  use_precision=off  precision=''  gain=1  offset=0  exp=1  use_mototune_group=off  mototune_group=motohawk_vardec_path(gcb)
      settings: SourceProductName=MotoHawk
  motohawk_probe21 : MotoHawk_lib/Calibration & Probing Blocks/motohawk_probe  nam='Coil_3'  show_more=off  name_source=Use Parameter  read_level=1  view_as=Number  enum_struct={'Disabled', 'Enabled'}  vector_style=Wide Row  use_help_units=off  help=''  units=''  use_header_enum=off  row_header_enum={}  col_header_enum={}  use_min_max=off  min_val=-inf  max_val=inf  use_precision=off  precision=''  gain=1  offset=0  exp=1  use_mototune_group=off  mototune_group=motohawk_vardec_path(gcb)
      settings: SourceProductName=MotoHawk
  motohawk_probe22 : MotoHawk_lib/Calibration & Probing Blocks/motohawk_probe  nam='Coil_4'  show_more=off  name_source=Use Parameter  read_level=1  view_as=Number  enum_struct={'Disabled', 'Enabled'}  vector_style=Wide Row  use_help_units=off  help=''  units=''  use_header_enum=off  row_header_enum={}  col_header_enum={}  use_min_max=off  min_val=-inf  max_val=inf  use_precision=off  precision=''  gain=1  offset=0  exp=1  use_mototune_group=off  mototune_group=motohawk_vardec_path(gcb)
      settings: SourceProductName=MotoHawk
  motohawk_pwm1 : MotoHawk_lib/Analog I//O Blocks/motohawk_pwm  res_name='E_Motor_Toruqe_Request'  text_resource=EST 1  target=ECU565-128  freq_mode=-1  min_freq=2  use_max_freq=off  max_freq=42949672.96  use_enable=off  use_brake=off  output_current=off  output_fault_status=off  use_child=off  use_vardec=off  nam='PWM'  read_level=1  write_level=1  group='System | I/O Pins | Outputs Config'
      settings: SourceProductName=MotoHawk
  wires:
  In10/1 -> motohawk_probe13/1, Saturation1/1
  Data Type Conversion8/1 -> motohawk_dout7/1
  Data Type Conversion7/1 -> motohawk_dout3/1
  Data Type Conversion6/1 -> motohawk_dout2/1
  Data Type Conversion5/1 -> motohawk_dout/1
  Data Type Conversion4/1 -> motohawk_dout1/1
  Data Type Conversion3/1 -> motohawk_dout4/1
  Data Type Conversion2/1 -> motohawk_dout6/1
  Data Type Conversion1/1 -> motohawk_dout5/1
  Data Type Conversion/1 -> motohawk_dout9/1
  In9/1 -> Data Type Conversion8/1, motohawk_probe22/1
  In8/1 -> Data Type Conversion7/1, motohawk_probe21/1
  In7/1 -> Data Type Conversion6/1, motohawk_probe20/1
  In6/1 -> Data Type Conversion5/1, motohawk_probe19/1
  motohawk_calibration15/1 -> Gain1/1
  Gain2/1 -> Data Type Conversion9/1
  Gain1/1 -> Data Type Conversion10/1
  In2/1 -> Data Type Conversion1/1, motohawk_probe15/1
  In5/1 -> Data Type Conversion4/1, motohawk_probe18/1
  In1/1 -> Data Type Conversion/1, motohawk_probe14/1
  In3/1 -> Data Type Conversion2/1, motohawk_probe16/1
  In4/1 -> Data Type Conversion3/1, motohawk_probe17/1
  Data Type Conversion9/1 -> motohawk_pwm1/1
  Data Type Conversion10/1 -> motohawk_pwm1/2
  Saturation1/1 -> Gain2/1

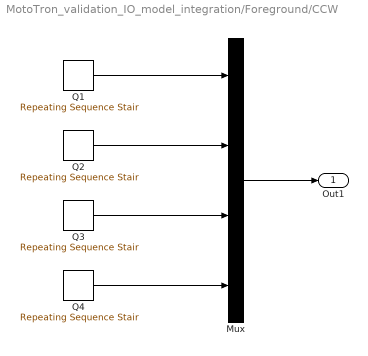
== system MotoTron_validation_IO_model_integration/Foreground/CCW ==
  Mux : Mux
  Q1 : simulink/Sources/Repeating Sequence Stair  OutValues=[1 0 0 0 0 0 1 1 1].'  tsamp=-1  OutMin=[]  OutMax=[]  OutDataTypeStr=double  OutputDataTypeScalingMode=double  OutDataType=fixdt(0,8)  ConRadixGroup=Best Precision: Vector-wise  OutScaling=2^-12
  Q2 : simulink/Sources/Repeating Sequence Stair  OutValues=[0 0 1 1 1 0 0 0 0].'  tsamp=-1  OutMin=[]  OutMax=[]  OutDataTypeStr=double  OutputDataTypeScalingMode=double  OutDataType=fixdt(0,8)  ConRadixGroup=Best Precision: Vector-wise  OutScaling=2^-12
  Q3 : simulink/Sources/Repeating Sequence Stair  OutValues=[1 1 1 0 0 0 0 0 1].'  tsamp=-1  OutMin=[]  OutMax=[]  OutDataTypeStr=double  OutputDataTypeScalingMode=double  OutDataType=fixdt(0,8)  ConRadixGroup=Best Precision: Vector-wise  OutScaling=2^-12
  Q4 : simulink/Sources/Repeating Sequence Stair  OutValues=[0 0 0 0 1 1 1 0 0].'  tsamp=-1  OutMin=[]  OutMax=[]  OutDataTypeStr=double  OutputDataTypeScalingMode=double  OutDataType=fixdt(0,8)  ConRadixGroup=Best Precision: Vector-wise  OutScaling=2^-12
  Out1 : Outport
  wires:
  Q1/1 -> Mux/1
  Q2/1 -> Mux/2
  Q3/1 -> Mux/3
  Q4/1 -> Mux/4
  Mux/1 -> Out1/1

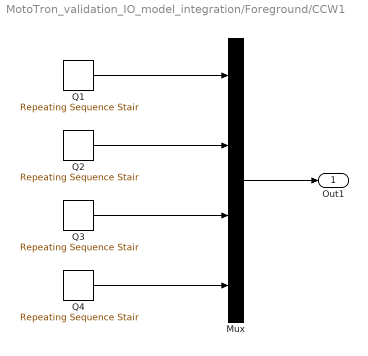
== system MotoTron_validation_IO_model_integration/Foreground/CCW1 ==
  Mux : Mux
  Q1 : simulink/Sources/Repeating Sequence Stair  OutValues=[1 0 0 0 0 0 1 1 1].'  tsamp=-1  OutMin=[]  OutMax=[]  OutDataTypeStr=double  OutputDataTypeScalingMode=double  OutDataType=fixdt(0,8)  ConRadixGroup=Best Precision: Vector-wise  OutScaling=2^-12
  Q2 : simulink/Sources/Repeating Sequence Stair  OutValues=[0 0 1 1 1 0 0 0 0].'  tsamp=-1  OutMin=[]  OutMax=[]  OutDataTypeStr=double  OutputDataTypeScalingMode=double  OutDataType=fixdt(0,8)  ConRadixGroup=Best Precision: Vector-wise  OutScaling=2^-12
  Q3 : simulink/Sources/Repeating Sequence Stair  OutValues=[1 1 1 0 0 0 0 0 1].'  tsamp=-1  OutMin=[]  OutMax=[]  OutDataTypeStr=double  OutputDataTypeScalingMode=double  OutDataType=fixdt(0,8)  ConRadixGroup=Best Precision: Vector-wise  OutScaling=2^-12
  Q4 : simulink/Sources/Repeating Sequence Stair  OutValues=[0 0 0 0 1 1 1 0 0].'  tsamp=-1  OutMin=[]  OutMax=[]  OutDataTypeStr=double  OutputDataTypeScalingMode=double  OutDataType=fixdt(0,8)  ConRadixGroup=Best Precision: Vector-wise  OutScaling=2^-12
  Out1 : Outport
  wires:
  Q1/1 -> Mux/1
  Q2/1 -> Mux/2
  Q3/1 -> Mux/3
  Q4/1 -> Mux/4
  Mux/1 -> Out1/1

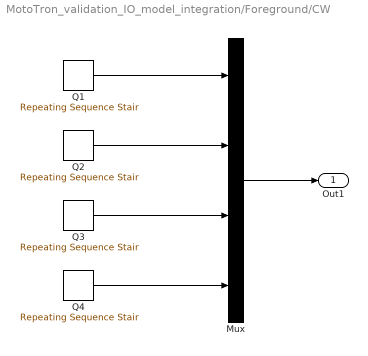
== system MotoTron_validation_IO_model_integration/Foreground/CW ==
  Mux : Mux
  Q1 : simulink/Sources/Repeating Sequence Stair  OutValues=[1 1 1 0 0 0 0 0 1].'  tsamp=-1  OutMin=[]  OutMax=[]  OutDataTypeStr=double  OutputDataTypeScalingMode=double  OutDataType=fixdt(0,8)  ConRadixGroup=Best Precision: Vector-wise  OutScaling=2^-12
  Q2 : simulink/Sources/Repeating Sequence Stair  OutValues=[0 0 0 0 1 1 1 0 0].'  tsamp=-1  OutMin=[]  OutMax=[]  OutDataTypeStr=double  OutputDataTypeScalingMode=double  OutDataType=fixdt(0,8)  ConRadixGroup=Best Precision: Vector-wise  OutScaling=2^-12
  Q3 : simulink/Sources/Repeating Sequence Stair  OutValues=[1 0 0 0 0 0 1 1 1].'  tsamp=-1  OutMin=[]  OutMax=[]  OutDataTypeStr=double  OutputDataTypeScalingMode=double  OutDataType=fixdt(0,8)  ConRadixGroup=Best Precision: Vector-wise  OutScaling=2^-12
  Q4 : simulink/Sources/Repeating Sequence Stair  OutValues=[0 0 1 1 1 0 0 0 0].'  tsamp=-1  OutMin=[]  OutMax=[]  OutDataTypeStr=double  OutputDataTypeScalingMode=double  OutDataType=fixdt(0,8)  ConRadixGroup=Best Precision: Vector-wise  OutScaling=2^-12
  Out1 : Outport
  wires:
  Mux/1 -> Out1/1
  Q4/1 -> Mux/4
  Q3/1 -> Mux/3
  Q2/1 -> Mux/2
  Q1/1 -> Mux/1

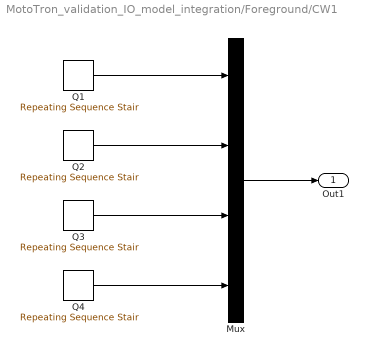
== system MotoTron_validation_IO_model_integration/Foreground/CW1 ==
  Mux : Mux
  Q1 : simulink/Sources/Repeating Sequence Stair  OutValues=[1 1 1 0 0 0 0 0 1].'  tsamp=-1  OutMin=[]  OutMax=[]  OutDataTypeStr=double  OutputDataTypeScalingMode=double  OutDataType=fixdt(0,8)  ConRadixGroup=Best Precision: Vector-wise  OutScaling=2^-12
  Q2 : simulink/Sources/Repeating Sequence Stair  OutValues=[0 0 0 0 1 1 1 0 0].'  tsamp=-1  OutMin=[]  OutMax=[]  OutDataTypeStr=double  OutputDataTypeScalingMode=double  OutDataType=fixdt(0,8)  ConRadixGroup=Best Precision: Vector-wise  OutScaling=2^-12
  Q3 : simulink/Sources/Repeating Sequence Stair  OutValues=[1 0 0 0 0 0 1 1 1].'  tsamp=-1  OutMin=[]  OutMax=[]  OutDataTypeStr=double  OutputDataTypeScalingMode=double  OutDataType=fixdt(0,8)  ConRadixGroup=Best Precision: Vector-wise  OutScaling=2^-12
  Q4 : simulink/Sources/Repeating Sequence Stair  OutValues=[0 0 1 1 1 0 0 0 0].'  tsamp=-1  OutMin=[]  OutMax=[]  OutDataTypeStr=double  OutputDataTypeScalingMode=double  OutDataType=fixdt(0,8)  ConRadixGroup=Best Precision: Vector-wise  OutScaling=2^-12
  Out1 : Outport
  wires:
  Mux/1 -> Out1/1
  Q4/1 -> Mux/4
  Q3/1 -> Mux/3
  Q2/1 -> Mux/2
  Q1/1 -> Mux/1
